simulink model "GravityModel"  (R2023b)
settings: Solver=FixedStepAuto  StartTime=0.0  StopTime=time.value  FixedStep=1  RelTol=1e-11  AbsTol=1e-12
undefined symbols (not defined in the file or in its folder): BeaconSpacecraft, Environment, MainSpacecraft, srp, thrust
libraries: dyn_lib x5, sensors_subsystems x4, nav_lib x1
settings Model: DataDictionary=SimulationDict.sldd  SimulationMode=accelerator  Creator=brent  LastModifiedBy=brent

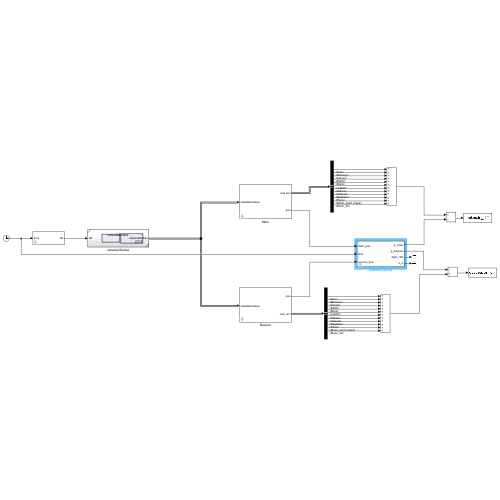
[thumbnail: Simulink's stored preview of the top-level diagram]
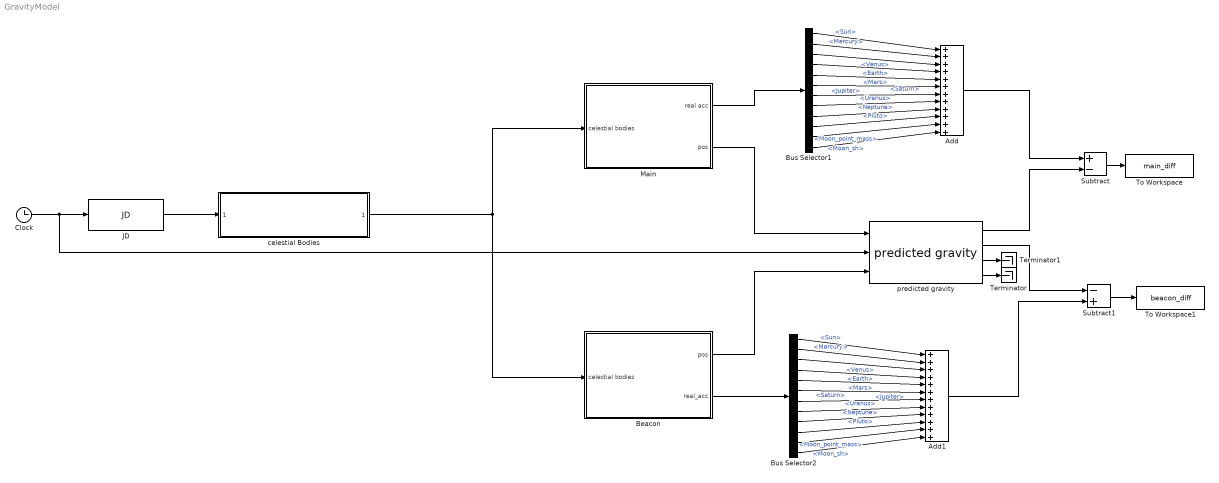
== system GravityModel ==
  Add : Sum  Inputs=++++++++++++
  Add1 : Sum  Inputs=++++++++++++
  Beacon : Subsystem  mask{Environment=Environment, Spacecraft=BeaconSpacecraft, sc_type="beacon"}
      mask prompts: Spacecraft "Spacecraft data"; sc_type "Spacecraft type"
  Bus Selector1 : BusSelector  OutputSignals=Sun,Mercury,Venus,Earth,Mars,Jupiter,Saturn,Uranus,Neptune,Pluto,Moon_point_mass,Moon_sh
  Bus Selector2 : BusSelector  OutputSignals=Sun,Mercury,Venus,Earth,Mars,Jupiter,Saturn,Uranus,Neptune,Pluto,Moon_point_mass,Moon_sh
  Clock : Clock
  JD : dyn_lib/JD  year=Environment.Date.year  month=Environment.Date.month  day=Environment.Date.day  hour=Environment.Date.hour  min=Environment.Date.min  sec=Environment.Date.sec
      settings: SourceProductName=Dynamics library
  Main : Subsystem  mask{Environment=Environment, Spacecraft=MainSpacecraft, sc_type="main"}
      mask prompts: Spacecraft "Spacecraft data"; sc_type "Spacecraft type"
  Subtract : Sum  Inputs=+-
  Subtract1 : Sum  Inputs=-+
  Terminator : Terminator
  Terminator1 : Terminator
  To Workspace : ToWorkspace  VariableName=main_diff  SampleTime=-1
  To Workspace1 : ToWorkspace  VariableName=beacon_diff  SampleTime=-1
  celestial Bodies : Subsystem  ReferencedSubsystem=celestialBodies
      settings: PermitHierarchicalResolution=None
  predicted gravity : nav_lib/predicted gravity  date=StartDate  Earth=Propagation.Earth  Moon=Propagation.Moon
      settings: SourceProductName=Navigation library
  wires:
  celestial Bodies/1 -> Beacon/1(celestial bodies), Main/1(celestial bodies)
  JD/1 -> celestial Bodies/1
  Clock/1 -> predicted gravity/2, JD/1
  Main/1(real acc) -> Bus Selector1/1
  Bus Selector1/1 -> Add/1  "<Sun>"
  Bus Selector1/2 -> Add/2  "<Mercury>"
  Bus Selector1/3 -> Add/3  "<Venus>"
  Bus Selector1/4 -> Add/4  "<Earth>"
  Bus Selector1/5 -> Add/5  "<Mars>"
  Bus Selector1/6 -> Add/6  "<Jupiter>"
  Bus Selector1/7 -> Add/7  "<Saturn>"
  Bus Selector1/8 -> Add/8  "<Uranus>"
  Bus Selector1/9 -> Add/9  "<Neptune>"
  Bus Selector1/10 -> Add/10  "<Pluto>"
  Bus Selector1/11 -> Add/11  "<Moon_point_mass>"
  Bus Selector1/12 -> Add/12  "<Moon_sh>"
  Bus Selector2/12 -> Add1/12  "<Moon_sh>"
  Bus Selector2/11 -> Add1/11  "<Moon_point_mass>"
  Bus Selector2/10 -> Add1/10  "<Pluto>"
  Bus Selector2/9 -> Add1/9  "<Neptune>"
  Bus Selector2/8 -> Add1/8  "<Uranus>"
  Bus Selector2/7 -> Add1/7  "<Saturn>"
  Bus Selector2/6 -> Add1/6  "<Jupiter>"
  Bus Selector2/5 -> Add1/5  "<Mars>"
  Bus Selector2/4 -> Add1/4  "<Earth>"
  Bus Selector2/3 -> Add1/3  "<Venus>"
  Bus Selector2/2 -> Add1/2  "<Mercury>"
  Bus Selector2/1 -> Add1/1  "<Sun>"
  Beacon/2(real_acc) -> Bus Selector2/1
  Beacon/1(pos) -> predicted gravity/3
  Main/2(pos) -> predicted gravity/1
  predicted gravity/4 -> Terminator/1
  predicted gravity/3 -> Terminator1/1
  Add/1 -> Subtract/1
  predicted gravity/1 -> Subtract/2
  Subtract/1 -> To Workspace/1
  predicted gravity/2 -> Subtract1/1
  Add1/1 -> Subtract1/2
  Subtract1/1 -> To Workspace1/1

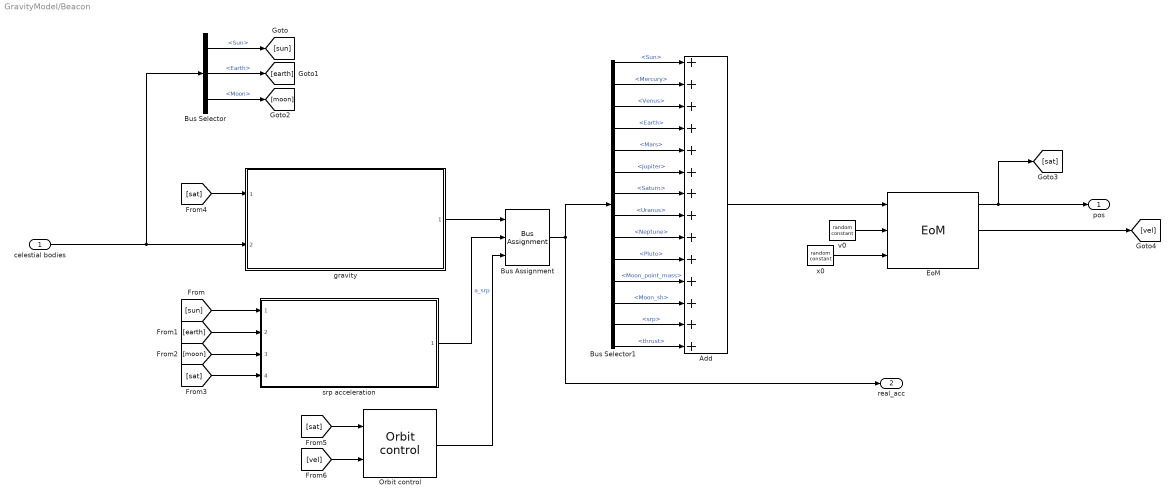
== system GravityModel/Beacon ==
  celestial bodies : Inport
  Add : Sum  Inputs=++++++++++++++
  Bus Assignment : BusAssignment  AssignedSignals=srp,thrust
  Bus Selector : BusSelector  OutputSignals=Sun,Earth,Moon
  Bus Selector1 : BusSelector  OutputSignals=Sun,Mercury,Venus,Earth,Mars,Jupiter,Saturn,Uranus,Neptune,Pluto,Moon_point_mass,Moon_sh,srp,thrust
  EoM : dyn_lib/EoM
      settings: SourceProductName=Dynamics library
  Orbit control : dyn_lib/Orbit control  VariantControl=Subsystem  flag=sc_type
      settings: SourceProductName=Dynamics library
  gravity : Subsystem  ReferencedSubsystem=gravitational_accelerations
  srp acceleration : Subsystem  ReferencedSubsystem=srp_acceleration  earth_radius=Environment.Earth.radius.value  sun_radius=Environment.Sun.radius.value  moon_radius=Environment.Moon.radius.value  C_R=Spacecraft.rp_coeff.value  A_sc=Spacecraft.radius.value^2*pi  m_sc=Spacecraft.mass.value  AU=Environment.AU.value  P=Environment.Sun.P.value
  v0 : sensors_subsystems/random constant  mean=Spacecraft.v0.nominal  dev=0
      settings: SourceProductName=Sensors library
  x0 : sensors_subsystems/random constant  mean=Spacecraft.x0.nominal  dev=0
      settings: SourceProductName=Sensors library
  pos : Outport
  real_acc : Outport  Port=2
  wires:
  [sat] -> srp acceleration/4
  EoM/2 -> [vel]
  Bus Selector1/6 -> Add/6  "<Jupiter>"
  gravity/1 -> Bus Assignment/1
  Bus Selector1/3 -> Add/3  "<Venus>"
  Bus Selector/1 -> [sun]  "<Sun>"
  Bus Selector1/12 -> Add/12  "<Moon_sh>"
  Bus Selector1/9 -> Add/9  "<Neptune>"
  x0/1 -> EoM/3
  Bus Selector1/14 -> Add/14  "<thrust>"
  Bus Selector1/5 -> Add/5  "<Mars>"
  Bus Selector1/8 -> Add/8  "<Uranus>"
  Bus Selector1/4 -> Add/4  "<Earth>"
  Bus Selector1/10 -> Add/10  "<Pluto>"
  Bus Selector1/7 -> Add/7  "<Saturn>"
  [earth] -> srp acceleration/2
  Orbit control/1 -> Bus Assignment/3
  Bus Assignment/1 -> Bus Selector1/1, real_acc/1
  Bus Selector1/13 -> Add/13  "<srp>"
  srp acceleration/1 -> Bus Assignment/2  "a_srp"
  [moon] -> srp acceleration/3
  Bus Selector1/11 -> Add/11  "<Moon_point_mass>"
  [sun] -> srp acceleration/1
  Bus Selector/3 -> [moon]  "<Moon>"
  Bus Selector1/2 -> Add/2  "<Mercury>"
  Add/1 -> EoM/1
  [vel] -> Orbit control/2
  celestial bodies/1 -> Bus Selector/1, gravity/2
  Bus Selector/2 -> [earth]  "<Earth>"
  [sat] -> Orbit control/1
  [sat] -> gravity/1
  Bus Selector1/1 -> Add/1  "<Sun>"
  v0/1 -> EoM/2
  EoM/1 -> pos/1, [sat]

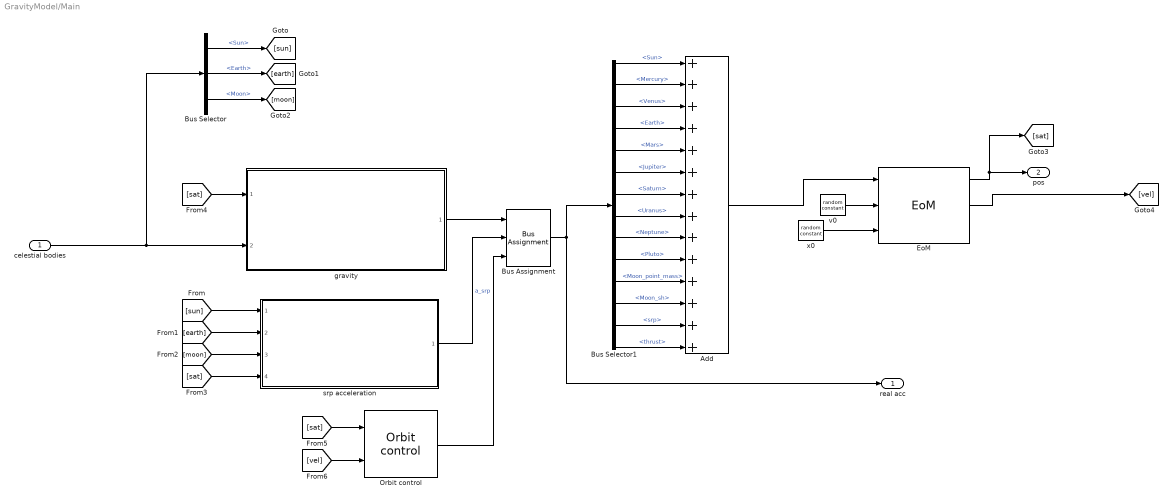
== system GravityModel/Main ==
  celestial bodies : Inport
  Add : Sum  Inputs=++++++++++++++
  Bus Assignment : BusAssignment  AssignedSignals=srp,thrust
  Bus Selector : BusSelector  OutputSignals=Sun,Earth,Moon
  Bus Selector1 : BusSelector  OutputSignals=Sun,Mercury,Venus,Earth,Mars,Jupiter,Saturn,Uranus,Neptune,Pluto,Moon_point_mass,Moon_sh,srp,thrust
  EoM : dyn_lib/EoM
      settings: SourceProductName=Dynamics library
  Orbit control : dyn_lib/Orbit control  VariantControl=Subsystem  flag=sc_type
      settings: SourceProductName=Dynamics library
  gravity : Subsystem  ReferencedSubsystem=gravitational_accelerations
  srp acceleration : Subsystem  ReferencedSubsystem=srp_acceleration  earth_radius=Environment.Earth.radius.value  sun_radius=Environment.Sun.radius.value  moon_radius=Environment.Moon.radius.value  C_R=Spacecraft.rp_coeff.value  A_sc=Spacecraft.radius.value^2*pi  m_sc=Spacecraft.mass.value  AU=Environment.AU.value  P=Environment.Sun.P.value
  v0 : sensors_subsystems/random constant  mean=Spacecraft.v0.nominal  dev=0
      settings: SourceProductName=Sensors library
  x0 : sensors_subsystems/random constant  mean=Spacecraft.x0.nominal  dev=0
      settings: SourceProductName=Sensors library
  real acc : Outport
  pos : Outport  Port=2
  wires:
  EoM/1 -> pos/1, [sat]
  v0/1 -> EoM/2
  Bus Selector1/1 -> Add/1  "<Sun>"
  [sat] -> gravity/1
  [sat] -> Orbit control/1
  Bus Selector/2 -> [earth]  "<Earth>"
  celestial bodies/1 -> gravity/2, Bus Selector/1
  [vel] -> Orbit control/2
  Add/1 -> EoM/1
  Bus Selector1/2 -> Add/2  "<Mercury>"
  Bus Selector/3 -> [moon]  "<Moon>"
  [sun] -> srp acceleration/1
  Bus Selector1/11 -> Add/11  "<Moon_point_mass>"
  [moon] -> srp acceleration/3
  srp acceleration/1 -> Bus Assignment/2  "a_srp"
  Bus Selector1/13 -> Add/13  "<srp>"
  Bus Assignment/1 -> real acc/1, Bus Selector1/1
  Orbit control/1 -> Bus Assignment/3
  [earth] -> srp acceleration/2
  Bus Selector1/7 -> Add/7  "<Saturn>"
  Bus Selector1/10 -> Add/10  "<Pluto>"
  Bus Selector1/4 -> Add/4  "<Earth>"
  Bus Selector1/8 -> Add/8  "<Uranus>"
  Bus Selector1/5 -> Add/5  "<Mars>"
  Bus Selector1/14 -> Add/14  "<thrust>"
  x0/1 -> EoM/3
  Bus Selector1/9 -> Add/9  "<Neptune>"
  Bus Selector1/12 -> Add/12  "<Moon_sh>"
  Bus Selector/1 -> [sun]  "<Sun>"
  Bus Selector1/3 -> Add/3  "<Venus>"
  gravity/1 -> Bus Assignment/1
  Bus Selector1/6 -> Add/6  "<Jupiter>"
  EoM/2 -> [vel]
  [sat] -> srp acceleration/4
